simulink model "arm_reference"  (R2024b)
settings: Solver=VariableStepAuto  StartTime=0.0  StopTime=200  RelTol=1e-3
libraries: models_lib x1
settings Model: Creator=ikostelidis  LastModifiedBy=ikostelidis

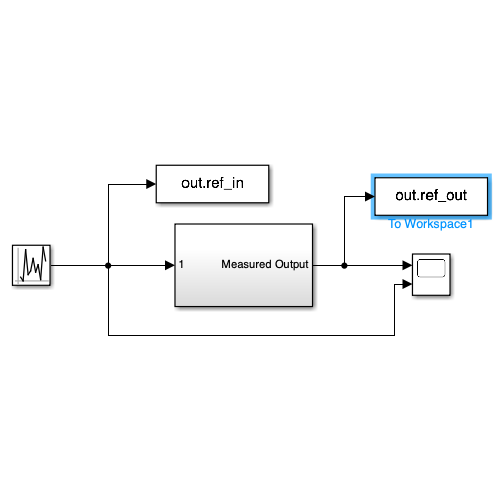
[thumbnail: Simulink's stored preview of the top-level diagram]
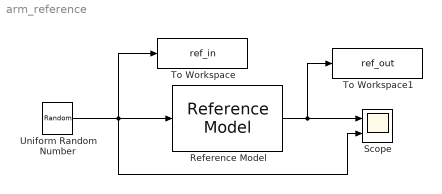
== system arm_reference ==
  Reference Model : models_lib/Reference Model  SystemSampleTime=-1  VariantActivationTime=update diagram  AllowFlexibleInterface=on  Latency=0  AutoFrameSizeCalculation=off
  Scope : Scope  NumInputPorts=2
  To Workspace : ToWorkspace  VariableName=ref_in  SampleTime=0.1
      settings: Save2DSignal=2-D array (concatenate along first dimension)
  To Workspace1 : ToWorkspace  VariableName=ref_out  SampleTime=0.1
      settings: Save2DSignal=2-D array (concatenate along first dimension)
  Uniform Random Number : UniformRandomNumber  Minimum=-4  Maximum=4  SampleTime=2
  wires:
  Uniform Random Number/1 -> Reference Model/1, Scope/2, To Workspace/1
  Reference Model/1 -> To Workspace1/1, Scope/1
